simulink library "Lib_EMTAT"  (R2023b)
settings: Solver=VariableStepAuto  StartTime=0.0  StopTime=10.0  RelTol=1e-3
undefined symbols (not defined in the file or in its folder): MWS
libraries: simulink x31, $bdroot x1
(part 4 of 4)

== system Lib_EMTAT/Components/Power Flow/Mechanical Shaft/Shaft Break Failure ==
  Failed? : Inport
  T : Inport  Port=2
  Constant : Constant  Value=0
  IsInf : RelationalOperator  Operator=isInf  OutDataTypeStr=boolean  RndMeth=Simplest  InputSameDT=off
  IsNaN : RelationalOperator  Operator=isNaN  OutDataTypeStr=boolean  RndMeth=Simplest  InputSameDT=off
  Logical Operator : Logic  Operator=OR  Inputs=3  AllPortsSameDT=off  OutDataTypeStr=boolean
  Switch : Switch  Criteria=u2 > Threshold  SaturateOnIntegerOverflow=off  InputSameDT=off
  "T " : Outport
  wires:
  Failed?/1 -> Logical Operator/1
  Constant/1 -> Switch/1
  T/1 -> IsNaN/1, IsInf/1, Switch/3
  Switch/1 -> "T "/1
  Logical Operator/1 -> Switch/2
  IsNaN/1 -> Logical Operator/2
  IsInf/1 -> Logical Operator/3

== system Lib_EMTAT/Components/Power Flow/Resistive Load Bank/Failure Determination ==
  Fail? : Inport
  OCFail : Outport
  wires:
  Fail?/1 -> OCFail/1

== system Lib_EMTAT/Components/Power Flow/Resistive Load Bank/Fix Divide By Zero. ==
  I^2 : Inport
  abs(Pset) : Inport  Port=2
  Constant : Constant  Value=eps
  Divide1 : Product  Inputs=/*
  If the square of the current is not equal to zero. : Switch  Criteria=u2 ~= 0  SaturateOnIntegerOverflow=off  InputSameDT=off
  R : Outport
  wires:
  Divide1/1 -> R/1
  abs(Pset)/1 -> Divide1/2
  I^2/1 -> If the square of the current is not equal to zero./2, If the square of the current is not equal to zero./1
  Constant/1 -> If the square of the current is not equal to zero./3
  If the square of the current is not equal to zero./1 -> Divide1/1

== system Lib_EMTAT/Components/Power Flow/Resistive Load Bank/Fix Divide By Zero.1 ==
  V : Inport
  Pset : Inport  Port=2
  Constant : Constant  Value=eps
  Divide1 : Product  Inputs=/*
  If voltage is not equal to zero. : Switch  Criteria=u2 ~= 0  SaturateOnIntegerOverflow=off  InputSameDT=off
  I : Outport
  wires:
  V/1 -> If voltage is not equal to zero./1, If voltage is not equal to zero./2
  Pset/1 -> Divide1/2
  Divide1/1 -> I/1
  Constant/1 -> If voltage is not equal to zero./3
  If voltage is not equal to zero./1 -> Divide1/1

== system Lib_EMTAT/Components/Power Flow/Resistive Load Bank/Open Circuit Failure - Line to Neutral Voltage ==
  Failed? : Inport
  I : Inport  Port=2
  Constant : Constant  Value=0
  IsInf : RelationalOperator  Operator=isInf  OutDataTypeStr=boolean  RndMeth=Simplest  InputSameDT=off
  IsNaN : RelationalOperator  Operator=isNaN  OutDataTypeStr=boolean  RndMeth=Simplest  InputSameDT=off
  Logical Operator : Logic  Operator=OR  Inputs=3  AllPortsSameDT=off  OutDataTypeStr=boolean
  Switch : Switch  Criteria=u2 > Threshold  SaturateOnIntegerOverflow=off  InputSameDT=off
  "I " : Outport
  wires:
  Failed?/1 -> Logical Operator/1
  Constant/1 -> Switch/1
  I/1 -> IsNaN/1, IsInf/1, Switch/3
  Switch/1 -> "I "/1
  Logical Operator/1 -> Switch/2
  IsNaN/1 -> Logical Operator/2
  IsInf/1 -> Logical Operator/3

== system Lib_EMTAT/Components/Power Flow/Supercapacitor/SOC ==
  Energy (W-h) : Inport
  Divide : Product  Inputs=*/
  Gain : Gain  Gain=100
  Total Stored Energy (W-h) : Constant  Value=TSE
  SOC : Outport
  wires:
  Gain/1 -> SOC/1
  Divide/1 -> Gain/1
  Total Stored Energy (W-h)/1 -> Divide/2
  Energy (W-h)/1 -> Divide/1

== system Lib_EMTAT/Components/Power Flow/Supercapacitor/Voltage, V to Energy, Wh ==
  V : Inport
  Gain2 : Gain  Gain=0.5*C
  J to Wh : Gain  Gain=0.000277778
  Square : Math  Operator=square
  E : Outport
  wires:
  V/1 -> Square/1
  Gain2/1 -> J to Wh/1
  Square/1 -> Gain2/1
  J to Wh/1 -> E/1

== system Lib_EMTAT/Components/Power Flow/Supercapacitor/Warnings ==
  SOC : Inport
  Compare To Constant : simulink/Logic and Bit Operations/Compare To Constant  relop=>  const=100  OutDataTypeStr=boolean
  Compare To Constant1 : simulink/Logic and Bit Operations/Compare To Constant  relop=<=  const=0  OutDataTypeStr=uint8
  Compare To Constant2 : simulink/Logic and Bit Operations/Compare To Constant  relop=<  const=2  OutDataTypeStr=boolean
  Logical Operator : Logic  AllPortsSameDT=off  OutDataTypeStr=boolean
  Memory : Memory
  SOC <= 0% : Subsystem
  SOC > 100% : Subsystem
  Sum : Sum  Inputs=|++
  wires:
  Logical Operator/1 -> SOC <= 0%/Trigger
  Compare To Constant2/1 -> Logical Operator/1
  Sum/1 -> Memory/1, Compare To Constant2/1
  Memory/1 -> Sum/2
  Compare To Constant1/1 -> Sum/1, Logical Operator/2
  Compare To Constant/1 -> SOC > 100%/Trigger
  SOC/1 -> Compare To Constant/1, Compare To Constant1/1

== system Lib_EMTAT/Components/Power Flow/Three Phase Electric Machine (Sink)/Compensate for Divide By Zero ==
  V_LN_rms : Inport
  PEquivElect : Inport  Port=2
  PF : Inport  Port=3
  Constant : Constant  Value=eps
  Constant1 : Constant  Value=3
  Divide : Product  Inputs=***
  Divide1 : Product  Inputs=/*
  Switch : Switch  Criteria=u2 ~= 0  SaturateOnIntegerOverflow=off  InputSameDT=off
  I_L_rms : Outport
  wires:
  Divide1/1 -> I_L_rms/1
  Constant/1 -> Switch/3
  Switch/1 -> Divide1/1
  Divide/1 -> Switch/2, Switch/1
  PEquivElect/1 -> Divide1/2
  Constant1/1 -> Divide/3
  V_LN_rms/1 -> Divide/2
  PF/1 -> Divide/1  "PF"

== system Lib_EMTAT/Components/Power Flow/Three Phase Electric Machine (Sink)/Direction Determination ==
  PMech : Inport
  Eff : Inport  Port=2
  Divide : Product  Inputs=/*
  Divide1 : Product  Inputs=**
  Switch : Switch  Criteria=u2 > Threshold  SaturateOnIntegerOverflow=off  InputSameDT=off
  PEquivElect : Outport
  wires:
  Switch/1 -> PEquivElect/1
  Eff/1 -> Divide1/2, Divide/1
  Divide1/1 -> Switch/3
  Divide/1 -> Switch/1
  PMech/1 -> Switch/2, Divide/2, Divide1/1

== system Lib_EMTAT/Components/Power Flow/Three Phase Electric Machine (Sink)/Efficiency ==
  T : Inport
  N : Inport  Port=2
  2-D Lookup Table : Lookup_n-D  BreakpointsForDimension1=X_C_SpeedVec_M  BreakpointsForDimension2=Y_C_TorqueVec_M  Table=T_C_EffArray_M  ExtrapMethod=Clip  UseLastTableValue=on  InternalRulePriority=Speed  RndMeth=Simplest
      settings: InputPortMap=u0,u1
  Abs : Abs  SaturateOnIntegerOverflow=off
  Abs1 : Abs  SaturateOnIntegerOverflow=off
  Eff : Outport
  wires:
  2-D Lookup Table/1 -> Eff/1
  N/1 -> Abs1/1
  Abs1/1 -> 2-D Lookup Table/1
  Abs/1 -> 2-D Lookup Table/2
  T/1 -> Abs/1

== system Lib_EMTAT/Components/Power Flow/Three Phase Electric Machine (Sink)/Failure Determination ==
  Fail? : Inport
  Compare To Constant : simulink/Logic and Bit Operations/Compare To Constant  relop===  const=1  OutDataTypeStr=boolean
  Compare To Constant1 : simulink/Logic and Bit Operations/Compare To Constant  relop===  const=2  OutDataTypeStr=boolean
  Data Type Conversion : DataTypeConversion  OutDataTypeStr=double  SaturateOnIntegerOverflow=off  RndMeth=Floor
  Data Type Conversion1 : DataTypeConversion  OutDataTypeStr=double  SaturateOnIntegerOverflow=off  RndMeth=Floor
  Failure Mode : Constant  Value=FM
  Logical Operator : Logic  AllPortsSameDT=off  OutDataTypeStr=boolean
  Logical Operator1 : Logic  AllPortsSameDT=off  OutDataTypeStr=boolean
  OCFail : Outport
  DegFail : Outport  Port=2
  wires:
  Data Type Conversion/1 -> OCFail/1
  Data Type Conversion1/1 -> DegFail/1
  Fail?/1 -> Logical Operator/2, Logical Operator1/2
  Logical Operator1/1 -> Data Type Conversion1/1
  Compare To Constant1/1 -> Logical Operator1/1
  Logical Operator/1 -> Data Type Conversion/1
  Compare To Constant/1 -> Logical Operator/1
  Failure Mode/1 -> Compare To Constant/1, Compare To Constant1/1

== system Lib_EMTAT/Components/Power Flow/Three Phase Electric Machine (Sink)/Open Circuit Failure - Line Current ==
  Failed? : Inport
  I_L_rms : Inport  Port=2
  Constant : Constant  Value=0
  IsInf : RelationalOperator  Operator=isInf  OutDataTypeStr=boolean  RndMeth=Simplest  InputSameDT=off
  IsNaN : RelationalOperator  Operator=isNaN  OutDataTypeStr=boolean  RndMeth=Simplest  InputSameDT=off
  Logical Operator : Logic  Operator=OR  Inputs=3  AllPortsSameDT=off  OutDataTypeStr=boolean
  Switch : Switch  Criteria=u2 > Threshold  SaturateOnIntegerOverflow=off  InputSameDT=off
  "I_L_rms " : Outport
  wires:
  IsInf/1 -> Logical Operator/3
  IsNaN/1 -> Logical Operator/2
  Logical Operator/1 -> Switch/2
  Switch/1 -> "I_L_rms "/1
  I_L_rms/1 -> Switch/3, IsInf/1, IsNaN/1
  Constant/1 -> Switch/1
  Failed?/1 -> Logical Operator/1

== system Lib_EMTAT/Components/Power Flow/Three Phase Electric Machine (Sink)/Open Circuit Failure - Torque ==
  Failed? : Inport
  T* : Inport  Port=2
  Constant : Constant  Value=0
  IsInf : RelationalOperator  Operator=isInf  OutDataTypeStr=boolean  RndMeth=Simplest  InputSameDT=off
  IsNaN : RelationalOperator  Operator=isNaN  OutDataTypeStr=boolean  RndMeth=Simplest  InputSameDT=off
  Logical Operator : Logic  Operator=OR  Inputs=3  AllPortsSameDT=off  OutDataTypeStr=boolean
  Switch : Switch  Criteria=u2 > Threshold  SaturateOnIntegerOverflow=off  InputSameDT=off
  "T  " : Outport
  wires:
  Failed?/1 -> Logical Operator/1
  Constant/1 -> Switch/1
  T*/1 -> IsNaN/1, IsInf/1, Switch/3
  Switch/1 -> "T  "/1
  Logical Operator/1 -> Switch/2
  IsNaN/1 -> Logical Operator/2
  IsInf/1 -> Logical Operator/3

== system Lib_EMTAT/Components/Power Flow/Three Phase Electric Machine (Sink)/Open Circuit Failure// Efficiency Scaling ==
  Eff : Inport
  DegFail? : Inport  Port=2
  OCFail? : Inport  Port=3
  HP : Inport  Port=4
  Constant : Constant  Value=0
  Constant1 : Constant
  Divide : Product  Inputs=**
  "If degradation failure, penalize Eff." : Switch  Criteria=u2 > Threshold  SaturateOnIntegerOverflow=off  InputSameDT=off
  "If open circuit failure, set Eff = 0." : Switch  Criteria=u2 > Threshold  SaturateOnIntegerOverflow=off  InputSameDT=off
  Sum : Sum  Inputs=+-|
  "Eff " : Outport
  wires:
  Sum/1 -> Divide/1
  Constant1/1 -> Sum/1
  Constant/1 -> "If open circuit failure, set Eff = 0."/1
  OCFail?/1 -> "If open circuit failure, set Eff = 0."/2
  "If open circuit failure, set Eff = 0."/1 -> "Eff "/1
  HP/1 -> Sum/2
  Divide/1 -> "If degradation failure, penalize Eff."/1
  Eff/1 -> "If degradation failure, penalize Eff."/3, Divide/2
  "If degradation failure, penalize Eff."/1 -> "If open circuit failure, set Eff = 0."/3
  DegFail?/1 -> "If degradation failure, penalize Eff."/2

== system Lib_EMTAT/Components/Power Flow/Three Phase Electric Machine (Sink)/Power Factor ==
  T : Inport
  N : Inport  Port=2
  2-D Lookup Table : Lookup_n-D  BreakpointsForDimension1=X_C_SpeedVec_M  BreakpointsForDimension2=Y_C_TorqueVec_M  Table=T_C_PFArray_M  ExtrapMethod=Clip  UseLastTableValue=on  InternalRulePriority=Speed  RndMeth=Simplest
      settings: InputPortMap=u0,u1
  Abs : Abs  SaturateOnIntegerOverflow=off
  Abs1 : Abs  SaturateOnIntegerOverflow=off
  PF : Outport
  wires:
  T/1 -> Abs/1
  Abs/1 -> 2-D Lookup Table/2
  Abs1/1 -> 2-D Lookup Table/1
  N/1 -> Abs1/1
  2-D Lookup Table/1 -> PF/1

== system Lib_EMTAT/Components/Power Flow/Three Phase Electric Machine (Source)/Compensate for Divide By Zero ==
  note: If Vin is not equal to zero, use its value.
      | If Vin is equal to zero, it will calculate a nan value for Iin. Set Iin to zero.
  PEquivMech : Inport
  N : Inport  Port=2
  Fix Divide By Zero. : Subsystem
  T : Outport
  wires:
  Fix Divide By Zero./1(T) -> T/1
  PEquivMech/1 -> Fix Divide By Zero./2(PEquivMech)
  N/1 -> Fix Divide By Zero./1(N)

== system Lib_EMTAT/Components/Power Flow/Three Phase Electric Machine (Source)/Direction Determination ==
  Eff : Inport
  Pelec : Inport  Port=2
  Divide3 : Product  Inputs=**
  Subsystem : Subsystem
  Switch : Switch  Criteria=u2 > Threshold  SaturateOnIntegerOverflow=off  InputSameDT=off
  PEquivMech : Outport
  wires:
  Subsystem/1(PEquivMech) -> Switch/3
  Switch/1 -> PEquivMech/1
  Eff/1 -> Divide3/1, Subsystem/2(Eff)
  Divide3/1 -> Switch/1
  Pelec/1 -> Divide3/2, Switch/2, Subsystem/1(Pelec)

== system Lib_EMTAT/Components/Power Flow/Three Phase Electric Machine (Source)/Efficiency ==
  T (lbf-ft) : Inport
  N (RPM) : Inport  Port=2
  2-D Lookup Table : Lookup_n-D  BreakpointsForDimension1=X_C_SpeedVec_M  BreakpointsForDimension2=Y_C_TorqueVec_M  Table=T_C_EffArray_M  ExtrapMethod=Clip  UseLastTableValue=on  InternalRulePriority=Speed  RndMeth=Simplest
      settings: InputPortMap=u0,u1
  Abs : Abs  SaturateOnIntegerOverflow=off
  Abs1 : Abs  SaturateOnIntegerOverflow=off
  Saturation : Saturate  UpperLimit=1  LowerLimit=eps
  Eff : Outport
  wires:
  Abs/1 -> 2-D Lookup Table/2
  T (lbf-ft)/1 -> Abs/1
  Saturation/1 -> Eff/1
  2-D Lookup Table/1 -> Saturation/1
  N (RPM)/1 -> Abs1/1
  Abs1/1 -> 2-D Lookup Table/1

== system Lib_EMTAT/Components/Power Flow/Three Phase Electric Machine (Source)/Failure Determination ==
  Fail? : Inport
  Compare To Constant : simulink/Logic and Bit Operations/Compare To Constant  relop===  const=1  OutDataTypeStr=boolean
  Compare To Constant1 : simulink/Logic and Bit Operations/Compare To Constant  relop===  const=2  OutDataTypeStr=boolean
  Data Type Conversion : DataTypeConversion  OutDataTypeStr=double  SaturateOnIntegerOverflow=off  RndMeth=Floor
  Data Type Conversion1 : DataTypeConversion  OutDataTypeStr=double  SaturateOnIntegerOverflow=off  RndMeth=Floor
  Failure Mode : Constant  Value=FM
  Logical Operator : Logic  AllPortsSameDT=off  OutDataTypeStr=boolean
  Logical Operator1 : Logic  AllPortsSameDT=off  OutDataTypeStr=boolean
  OCFail : Outport
  DegFail : Outport  Port=2
  wires:
  Data Type Conversion/1 -> OCFail/1
  Data Type Conversion1/1 -> DegFail/1
  Fail?/1 -> Logical Operator/2, Logical Operator1/2
  Logical Operator1/1 -> Data Type Conversion1/1
  Compare To Constant1/1 -> Logical Operator1/1
  Logical Operator/1 -> Data Type Conversion/1
  Compare To Constant/1 -> Logical Operator/1
  Failure Mode/1 -> Compare To Constant/1, Compare To Constant1/1

== system Lib_EMTAT/Components/Power Flow/Three Phase Electric Machine (Source)/Open Circuit Failure - Line-Neutral Voltage ==
  Failed? : Inport
  V_LN_rms : Inport  Port=2
  Constant : Constant  Value=0
  IsInf : RelationalOperator  Operator=isInf  OutDataTypeStr=boolean  RndMeth=Simplest  InputSameDT=off
  IsNaN : RelationalOperator  Operator=isNaN  OutDataTypeStr=boolean  RndMeth=Simplest  InputSameDT=off
  Logical Operator : Logic  Operator=OR  Inputs=3  AllPortsSameDT=off  OutDataTypeStr=boolean
  Switch : Switch  Criteria=u2 > Threshold  SaturateOnIntegerOverflow=off  InputSameDT=off
  "V_LN_rms " : Outport
  wires:
  IsInf/1 -> Logical Operator/3
  IsNaN/1 -> Logical Operator/2
  Logical Operator/1 -> Switch/2
  Switch/1 -> "V_LN_rms "/1
  V_LN_rms/1 -> Switch/3, IsInf/1, IsNaN/1
  Constant/1 -> Switch/1
  Failed?/1 -> Logical Operator/1

== system Lib_EMTAT/Components/Power Flow/Three Phase Electric Machine (Source)/Open Circuit// Degradation Failure ==
  Eff : Inport
  DegFail? : Inport  Port=2
  OCFail? : Inport  Port=3
  HP : Inport  Port=4
  Constant : Constant  Value=0
  Constant1 : Constant
  Divide : Product  Inputs=**
  "If degradation failure, penalize Eff." : Switch  Criteria=u2 > Threshold  SaturateOnIntegerOverflow=off  InputSameDT=off
  "If open circuit failure, set Eff = 0." : Switch  Criteria=u2 > Threshold  SaturateOnIntegerOverflow=off  InputSameDT=off
  Sum : Sum  Inputs=+-|
  "Eff " : Outport
  wires:
  Sum/1 -> Divide/1
  Constant1/1 -> Sum/1
  Constant/1 -> "If open circuit failure, set Eff = 0."/1
  OCFail?/1 -> "If open circuit failure, set Eff = 0."/2
  "If open circuit failure, set Eff = 0."/1 -> "Eff "/1
  HP/1 -> Sum/2
  Divide/1 -> "If degradation failure, penalize Eff."/1
  Eff/1 -> "If degradation failure, penalize Eff."/3, Divide/2
  "If degradation failure, penalize Eff."/1 -> "If open circuit failure, set Eff = 0."/3
  DegFail?/1 -> "If degradation failure, penalize Eff."/2

== system Lib_EMTAT/Components/Power Flow/AC-AC Transformer (Efficiency Map)/Compensate for Divide By Zero/Fix Divide By Zero. ==
  V_LN_rms_1 : Inport
  P_AC_1 : Inport  Port=2
  Constant1 : Constant  Value=eps  SampleTime=-1
  Divide1 : Product  Inputs=/*
  Switch1 : Switch  Criteria=u2 ~= 0  SaturateOnIntegerOverflow=off  InputSameDT=off
  I_L_rms_1 : Outport
  wires:
  Switch1/1 -> Divide1/1
  Constant1/1 -> Switch1/3
  V_LN_rms_1/1 -> Switch1/1, Switch1/2
  P_AC_1/1 -> Divide1/2
  Divide1/1 -> I_L_rms_1/1

== system Lib_EMTAT/Components/Power Flow/AC-AC Transformer (Power Loss Map)/Compensate for Divide By Zero/Fix Divide By Zero. ==
  V_LN_rms_1 : Inport
  P_AC_1 : Inport  Port=2
  Constant1 : Constant  Value=eps  SampleTime=-1
  Divide1 : Product  Inputs=/*
  Switch1 : Switch  Criteria=u2 ~= 0  SaturateOnIntegerOverflow=off  InputSameDT=off
  I_L_rms_1 : Outport
  wires:
  Divide1/1 -> I_L_rms_1/1
  P_AC_1/1 -> Divide1/2
  V_LN_rms_1/1 -> Switch1/2, Switch1/1
  Constant1/1 -> Switch1/3
  Switch1/1 -> Divide1/1

== system Lib_EMTAT/Components/Power Flow/AC-AC Transformer (Power Loss Map)/Efficiency/Fix Divide By Zero. ==
  abs(P_AC_2) : Inport
  abs(P_AC_1) : Inport  Port=2
  Constant1 : Constant  Value=eps  SampleTime=-1
  Divide1 : Product  Inputs=/*
  Switch1 : Switch  Criteria=u2 ~= 0  SaturateOnIntegerOverflow=off  InputSameDT=off
  Eff : Outport
  wires:
  abs(P_AC_2)/1 -> Switch1/2, Switch1/1
  abs(P_AC_1)/1 -> Divide1/2
  Divide1/1 -> Eff/1
  Constant1/1 -> Switch1/3
  Switch1/1 -> Divide1/1

== system Lib_EMTAT/Components/Power Flow/AC-AC Transformer (Power Loss Map)/Efficiency/Fix Divide By Zero.1 ==
  abs(P_AC_1) : Inport
  abs(P_AC_2) : Inport  Port=2
  Constant1 : Constant  Value=eps  SampleTime=-1
  Divide1 : Product  Inputs=/*
  Switch1 : Switch  Criteria=u2 ~= 0  SaturateOnIntegerOverflow=off  InputSameDT=off
  Eff : Outport
  wires:
  Divide1/1 -> Eff/1
  abs(P_AC_1)/1 -> Switch1/2, Switch1/1
  abs(P_AC_2)/1 -> Divide1/2
  Constant1/1 -> Switch1/3
  Switch1/1 -> Divide1/1

== system Lib_EMTAT/Components/Power Flow/AC-DC Rectifier (Power Loss Map)/Efficiency/Fix Divide By Zero. ==
  abs(P_AC) : Inport
  abs(P_DC) : Inport  Port=2
  Constant : Constant  Value=eps
  Divide1 : Product  Inputs=/*
  Switch : Switch  Criteria=u2 ~= 0  SaturateOnIntegerOverflow=off  InputSameDT=off
  Eff : Outport
  wires:
  abs(P_DC)/1 -> Divide1/2
  Divide1/1 -> Eff/1
  Constant/1 -> Switch/3
  abs(P_AC)/1 -> Switch/2, Switch/1
  Switch/1 -> Divide1/1

== system Lib_EMTAT/Components/Power Flow/AC-DC Rectifier (Power Loss Map)/Efficiency/Fix Divide By Zero.1 ==
  abs(P_DC) : Inport
  abs(P_AC) : Inport  Port=2
  Constant1 : Constant  Value=eps
  Divide1 : Product  Inputs=/*
  Switch1 : Switch  Criteria=u2 ~= 0  SaturateOnIntegerOverflow=off  InputSameDT=off
  Eff : Outport
  wires:
  Divide1/1 -> Eff/1
  abs(P_AC)/1 -> Divide1/2
  Constant1/1 -> Switch1/3
  abs(P_DC)/1 -> Switch1/2, Switch1/1
  Switch1/1 -> Divide1/1

== system Lib_EMTAT/Components/Power Flow/DC-AC Inverter (Efficiency Map)/Compensate for Divide By Zero/Fix Divide By Zero. ==
  V_DC : Inport
  PEquivDC : Inport  Port=2
  Constant1 : Constant  Value=eps
  Divide1 : Product  Inputs=/*
  Switch1 : Switch  Criteria=u2 ~= 0  SaturateOnIntegerOverflow=off  InputSameDT=off
  I_DC : Outport
  wires:
  Switch1/1 -> Divide1/1
  Constant1/1 -> Switch1/3
  V_DC/1 -> Switch1/1, Switch1/2
  Divide1/1 -> I_DC/1
  PEquivDC/1 -> Divide1/2

== system Lib_EMTAT/Components/Power Flow/DC-AC Inverter (Power Loss Map)/Compensate for Divide By Zero/Fix Divide By Zero. ==
  V_DC : Inport
  PEquivDC : Inport  Port=2
  Constant1 : Constant  Value=eps
  Divide1 : Product  Inputs=/*
  Switch1 : Switch  Criteria=u2 ~= 0  SaturateOnIntegerOverflow=off  InputSameDT=off
  I_DC : Outport
  wires:
  PEquivDC/1 -> Divide1/2
  Divide1/1 -> I_DC/1
  V_DC/1 -> Switch1/2, Switch1/1
  Constant1/1 -> Switch1/3
  Switch1/1 -> Divide1/1

== system Lib_EMTAT/Components/Power Flow/DC-AC Inverter (Power Loss Map)/Efficiency/Fix Divide By Zero. ==
  abs(P_AC) : Inport
  abs(P_DC) : Inport  Port=2
  Constant : Constant  Value=eps
  Divide1 : Product  Inputs=/*
  Switch : Switch  Criteria=u2 ~= 0  SaturateOnIntegerOverflow=off  InputSameDT=off
  Eff : Outport
  wires:
  abs(P_DC)/1 -> Divide1/2
  Divide1/1 -> Eff/1
  Constant/1 -> Switch/3
  abs(P_AC)/1 -> Switch/2, Switch/1
  Switch/1 -> Divide1/1

== system Lib_EMTAT/Components/Power Flow/DC-AC Inverter (Power Loss Map)/Efficiency/Fix Divide By Zero.1 ==
  abs(P_DC) : Inport
  abs(P_AC) : Inport  Port=2
  Constant1 : Constant  Value=eps
  Divide1 : Product  Inputs=/*
  Switch1 : Switch  Criteria=u2 ~= 0  SaturateOnIntegerOverflow=off  InputSameDT=off
  Eff : Outport
  wires:
  Divide1/1 -> Eff/1
  abs(P_AC)/1 -> Divide1/2
  Constant1/1 -> Switch1/3
  abs(P_DC)/1 -> Switch1/2, Switch1/1
  Switch1/1 -> Divide1/1

== system Lib_EMTAT/Components/Power Flow/DC-DC Converter (Efficiency Map) (Regulate Output Voltage)/Compensate for Divide By Zero/Fix Divide By Zero. ==
  Vin : Inport
  Pin : Inport  Port=2
  Constant : Constant  Value=eps
  Divide1 : Product  Inputs=/*
  Switch : Switch  Criteria=u2 ~= 0  SaturateOnIntegerOverflow=off  InputSameDT=off
  Iin : Outport
  wires:
  Switch/1 -> Divide1/1
  Divide1/1 -> Iin/1
  Constant/1 -> Switch/3
  Vin/1 -> Switch/2, Switch/1
  Pin/1 -> Divide1/2

== system Lib_EMTAT/Components/Power Flow/DC-DC Converter (Efficiency Map) (Set Output Voltage)/Compensate for Divide By Zero/Fix Divide By Zero. ==
  Vin : Inport
  Pin : Inport  Port=2
  Constant : Constant  Value=eps  SampleTime=-1
  Divide1 : Product  Inputs=/*
  Switch : Switch  Criteria=u2 ~= 0  SaturateOnIntegerOverflow=off  InputSameDT=off
  Iin : Outport
  wires:
  Switch/1 -> Divide1/1
  Vin/1 -> Switch/1, Switch/2
  Constant/1 -> Switch/3
  Divide1/1 -> Iin/1
  Pin/1 -> Divide1/2

== system Lib_EMTAT/Components/Power Flow/DC-DC Converter (Power Loss Map) (Regulate Output Voltage)/Compensate for Divide By Zero/Fix Divide By Zero. ==
  Vin : Inport
  Pin : Inport  Port=2
  Constant : Constant  Value=eps
  Divide1 : Product  Inputs=/*
  Switch : Switch  Criteria=u2 ~= 0  SaturateOnIntegerOverflow=off  InputSameDT=off
  Iin : Outport
  wires:
  Pin/1 -> Divide1/2
  Vin/1 -> Switch/1, Switch/2
  Constant/1 -> Switch/3
  Divide1/1 -> Iin/1
  Switch/1 -> Divide1/1

== system Lib_EMTAT/Components/Power Flow/DC-DC Converter (Power Loss Map) (Regulate Output Voltage)/Efficiency/Fix Divide By Zero. ==
  abs(Pout) : Inport
  abs(Pin) : Inport  Port=2
  Constant1 : Constant  Value=eps
  Divide1 : Product  Inputs=/*
  Switch1 : Switch  Criteria=u2 ~= 0  SaturateOnIntegerOverflow=off  InputSameDT=off
  Eff : Outport
  wires:
  abs(Pin)/1 -> Divide1/2
  Divide1/1 -> Eff/1
  abs(Pout)/1 -> Switch1/2, Switch1/1
  Constant1/1 -> Switch1/3
  Switch1/1 -> Divide1/1

== system Lib_EMTAT/Components/Power Flow/DC-DC Converter (Power Loss Map) (Regulate Output Voltage)/Efficiency/Fix Divide By Zero.1 ==
  abs(Pin) : Inport
  abs(Pout) : Inport  Port=2
  Constant : Constant  Value=eps
  Divide1 : Product  Inputs=/*
  Switch : Switch  Criteria=u2 ~= 0  SaturateOnIntegerOverflow=off  InputSameDT=off
  Eff : Outport
  wires:
  abs(Pout)/1 -> Divide1/2
  abs(Pin)/1 -> Switch/2, Switch/1
  Constant/1 -> Switch/3
  Divide1/1 -> Eff/1
  Switch/1 -> Divide1/1

== system Lib_EMTAT/Components/Power Flow/DC-DC Converter (Power Loss Map) (Set Output Voltage)/Compensate for Divide By Zero/Fix Divide By Zero. ==
  Vin : Inport
  Pin : Inport  Port=2
  Constant : Constant  Value=eps  SampleTime=-1
  Divide1 : Product  Inputs=/*
  Switch : Switch  Criteria=u2 ~= 0  SaturateOnIntegerOverflow=off  InputSameDT=off
  Iin : Outport
  wires:
  Pin/1 -> Divide1/2
  Divide1/1 -> Iin/1
  Constant/1 -> Switch/3
  Vin/1 -> Switch/2, Switch/1
  Switch/1 -> Divide1/1

== system Lib_EMTAT/Components/Power Flow/DC-DC Converter (Power Loss Map) (Set Output Voltage)/Efficiency/Fix Divide By Zero. ==
  abs(Pout) : Inport
  abs(Pin) : Inport  Port=2
  Constant1 : Constant  Value=eps
  Divide1 : Product  Inputs=/*
  Switch1 : Switch  Criteria=u2 ~= 0  SaturateOnIntegerOverflow=off  InputSameDT=off
  Eff : Outport
  wires:
  Divide1/1 -> Eff/1
  abs(Pin)/1 -> Divide1/2
  Constant1/1 -> Switch1/3
  abs(Pout)/1 -> Switch1/2, Switch1/1
  Switch1/1 -> Divide1/1

== system Lib_EMTAT/Components/Power Flow/DC-DC Converter (Power Loss Map) (Set Output Voltage)/Efficiency/Fix Divide By Zero.1 ==
  abs(Pin) : Inport
  abs(Pout) : Inport  Port=2
  Constant : Constant  Value=eps
  Divide1 : Product  Inputs=/*
  Switch : Switch  Criteria=u2 ~= 0  SaturateOnIntegerOverflow=off  InputSameDT=off
  Eff : Outport
  wires:
  abs(Pin)/1 -> Switch/1, Switch/2
  abs(Pout)/1 -> Divide1/2
  Constant/1 -> Switch/3
  Divide1/1 -> Eff/1
  Switch/1 -> Divide1/1

== system Lib_EMTAT/Components/Power Flow/Supercapacitor/Warnings/SOC <= 0% ==
  Trigger : TriggerPort  VariantControl=(inherit)
  MATLAB Function : MATLAB Function  TreatAsAtomicUnit=on

== system Lib_EMTAT/Components/Power Flow/Supercapacitor/Warnings/SOC > 100% ==
  Trigger : TriggerPort  VariantControl=(inherit)
  MATLAB Function : MATLAB Function  TreatAsAtomicUnit=on

== system Lib_EMTAT/Components/Power Flow/Three Phase Electric Machine (Source)/Compensate for Divide By Zero/Fix Divide By Zero. ==
  N : Inport
  PEquivMech : Inport  Port=2
  Constant : Constant  Value=eps
  Divide1 : Product  Inputs=/*
  Switch : Switch  Criteria=u2 ~= 0  SaturateOnIntegerOverflow=off  InputSameDT=off
  T : Outport
  wires:
  PEquivMech/1 -> Divide1/2
  Divide1/1 -> T/1
  Constant/1 -> Switch/3
  N/1 -> Switch/2, Switch/1
  Switch/1 -> Divide1/1

== system Lib_EMTAT/Components/Power Flow/Three Phase Electric Machine (Source)/Direction Determination/Subsystem ==
  Pelec : Inport
  Eff : Inport  Port=2
  Constant : Constant  Value=0
  Divide : Product  Inputs=**
  Divide2 : Product  Inputs=*/
  Switch : Switch  Criteria=u2 ~= 0  SaturateOnIntegerOverflow=off  InputSameDT=off
  PEquivMech : Outport
  wires:
  Switch/1 -> PEquivMech/1
  Pelec/1 -> Divide2/1
  Divide2/1 -> Switch/1
  Eff/1 -> Divide2/2, Switch/2, Divide/2
  Divide/1 -> Switch/3
  Constant/1 -> Divide/1

== matlab function Lib_EMTAT/Components/Power Flow/Supercapacitor/Warnings/SOC <= 0%/MATLAB Function ==
  data: BlkNm parameter
function fcn(BlkNm)
disp(['Warning in ' BlkNm ': State of charge is 0 percent.']);
end

== matlab function Lib_EMTAT/Components/Power Flow/Supercapacitor/Warnings/SOC > 100%/MATLAB Function ==
  data: BlkNm parameter
function fcn(BlkNm)
disp(['Warning in ' BlkNm ': State of charge is greater than 100 percent.']);
end

== matlab function Lib_EMTAT/Components/Power Flow/Electrical Bus/MATLAB Function ==
  data: u input; y output double; Nb parameter
function y = sumBranches(u,Nb)
if length(u)~=Nb
    yi = zeros(Nb,1); %initialize vector in for loop.
    for i = 1:1:length(u)/Nb
        yi(i) = sum(u(i:Nb:length(u)));
    end
else
    yi = sum(u);
end
y = yi;

== matlab function Lib_EMTAT/Components/Power Flow/Power Supply (Set Voltage)/MATLAB Function ==
  data: u input; y output double; Nb parameter
function y = sumBranches(u,Nb)
if length(u)~=Nb
    yi = zeros(Nb,1); %initialize vector in for loop.
    for i = 1:1:length(u)/Nb
        yi(i) = sum(u(i:Nb:length(u)));
    end
else
    yi = sum(u);
end
y = yi;

== matlab function Lib_EMTAT/Components/Power Flow/Current Junction/MATLAB Function ==
  data: u input; y output double; Nb parameter
function y = sumBranches(u,Nb)
yi = zeros(Nb,1); %initialize vector in for loop.
if Nb == 1
    yi = sum(u);
else
    for i = 0:1:Nb-1
        yi(i+1) = sum(u(i*Nb+1:i*Nb+Nb));
    end
end
y = yi;

== matlab function Lib_EMTAT/Components/Power Flow/Current Distribution/MATLAB Function ==
  data: I input; Isplit output double; Idmd input
function Isplit = splitBranches1(I, Idmd)

yi = zeros(length(Idmd),1); %initialize vector in for loop.
if length(I) == length(Idmd)
    yi = I.*Idmd./sum(Idmd);
else
    for i = 1:1:length(I)

            yi(i*length(I)-length(I)+1:i*length(I),1) = I(i).*Idmd(i*length(I)-length(I)+1:i*length(I))./sum(Idmd(i*length(I)-length(I)+1: i*length(I)));
    end
end
Isplit = yi;
